simulink model "ship_5_5e"  (R2018a)
settings: Solver=VariableStepAuto  StartTime=0.0  StopTime=8000  RelTol=1e-3  EnableMultiTasking=on
values from neighbouring files (symbols this model uses):
  Kpd = sqrt(Tf^2*omegac^4+omegac^2)/K    [oppg5_3.m]    (also in oppg5_5.m = 0.8159)
  Td = T    (= 75)    [oppg5_3.m]    (also in oppg5_5.m)
  Tf = -1/(omegac*tand(130))    [oppg5_3.m]    (also in oppg5_5.m = 8.391)
libraries: simulink x1
settings Model: Creator=markh  LastModifiedBy=mariu
settings DataIOCC: LimitDataPoints=on  MaxDataPoints=100000  SaveFormat=Array  SignalLoggingSaveFormat=ModelDataLogs  SignalLoggingName=sigsOut
settings OptimizationCC: InitFltsAndDblsToZero=on  LifeSpan=inf
settings DebuggingCC: SaveWithParameterizedLinksMsg=none  UnderspecifiedInitializationDetection=Classic  MergeDetectMultiDrivingBlocksExec=none  SignalResolutionControl=TryResolveAllWithWarning  MultiTaskDSMMsg=warning  MultiTaskCondExecSysMsg=none  FcnCallInpInsideContextMsg=warning  StateNameClashWarn=warning  SFUnexpectedBacktrackingDiag=warning  SFNoUnconditionalDefaultTransitionDiag=warning  SFExecutionAtInitializationDiag=none
settings HardwareCC: ProdBitPerPointer=32  ProdBitPerSizeT=32  ProdBitPerPtrDiffT=32  ProdLargestAtomicFloat=None  ProdIntDivRoundTo=Undefined  ProdEndianess=Unspecified  ProdWordSize=32  ProdHWDeviceType=32-bit Generic  TargetUnknown=on
settings ModelReferenceCC: PropagateSignalLabelsOutOfModel=off
settings RTWCC: Description=Generic Real-Time Target
settings CodeAppCC: StateflowObjectComments=on
settings GRTTargetCC: TargetFcnLib=ansi_tfl_tmw.mat  TargetLangStandard=C89/C90 (ANSI)  GeneratePreprocessorConditionals=Disable all  CombineOutputUpdateFcns=off  GRTInterface=on
settings ConfigComp: CovMetricSettings=dw  CovHtmlReporting=on  CovSaveCumulativeToWorkspaceVar=on  CovSaveSingleToWorkspaceVar=on  CovExternalEMLEnable=off

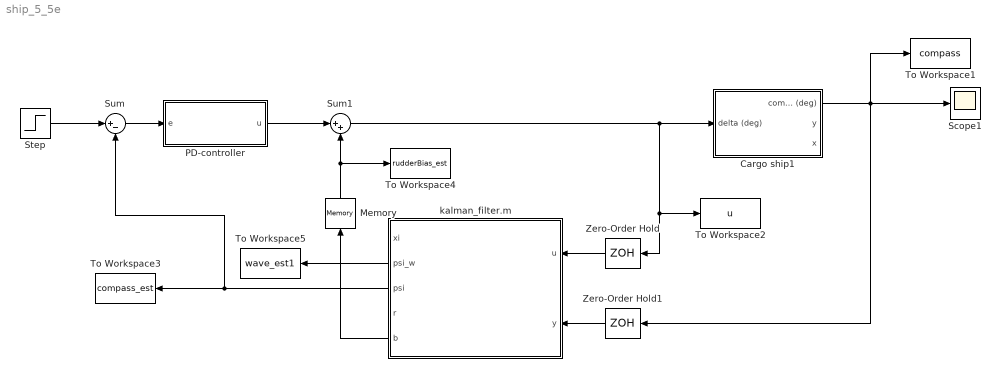
== system ship_5_5e ==
  " kalman_filter.m" : MATLAB Function  TreatAsAtomicUnit=on
  Cargo ship1 : Subsystem  mask(Simple shipmodel for a cargo ship){noise=on, current=on, logic=on}
      mask prompts: noise "measurement noise"; logic "waves"
      mask help:
      | Measurement noise:
      | 	checked = noise on
      | 	unchecked = noise off
      |
      | Current:
      | 	checked = current on
      | 	unchecked = current off
      |
      | Waves:
      | 	checked = waves on
      | 	unchecked = waves off
      |
      | Author: Jørgen Spjøtvold, 9/10-2003
      | TTK 4115 Linear system theory.
      | Modified by Jostein Bakkeheim 26/10-2006
  Memory : Memory
  PD-controller : Subsystem
  Scope1 : Scope
  Step : Step  Time=0  After=30  SampleTime=0
  Sum : Sum  Inputs=|+-
  Sum1 : Sum  Inputs=|++
  To Workspace1 : ToWorkspace  VariableName=compass  SaveFormat=Timeseries  SampleTime=-1
  To Workspace2 : ToWorkspace  VariableName=u  SaveFormat=Timeseries  SampleTime=-1
  To Workspace3 : ToWorkspace  VariableName=compass_est  SaveFormat=Timeseries  SampleTime=-1
  To Workspace4 : ToWorkspace  VariableName=rudderBias_est  SaveFormat=Timeseries  SampleTime=-1
  To Workspace5 : ToWorkspace  VariableName=wave_est1  SaveFormat=Timeseries  SampleTime=-1
  Zero-Order Hold : ZeroOrderHold  SampleTime=0.1
  Zero-Order Hold1 : ZeroOrderHold  SampleTime=0.1
  wires:
  Cargo ship1/1(compass (deg)) -> Zero-Order Hold1/1, To Workspace1/1, Scope1/1
  Sum/1 -> PD-controller/1(e)
  Zero-Order Hold1/1 -> " kalman_filter.m"/2(y)
  Zero-Order Hold/1 -> " kalman_filter.m"/1(u)
  " kalman_filter.m"/3(psi) -> Sum/2, To Workspace3/1
  PD-controller/1(u) -> Sum1/1
  Sum1/1 -> To Workspace2/1, Zero-Order Hold/1, Cargo ship1/1(delta (deg))
  " kalman_filter.m"/5(b) -> Memory/1
  Memory/1 -> To Workspace4/1, Sum1/2
  Step/1 -> Sum/1
  " kalman_filter.m"/2(psi_w) -> To Workspace5/1

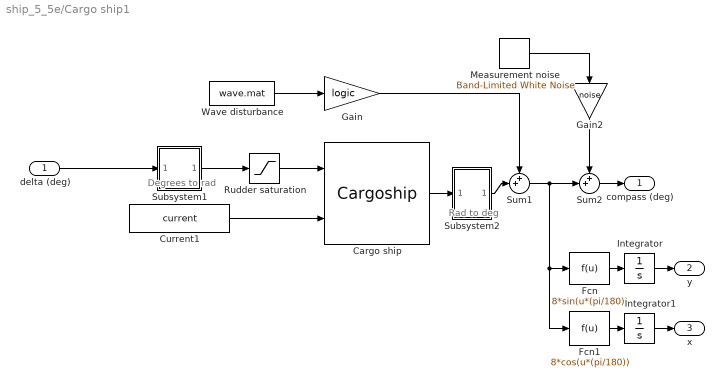
== system ship_5_5e/Cargo ship1 ==
  note: Degrees to rad
  note: Rad to deg
  delta (deg) : Inport
  Cargo ship : S-Function  FunctionName=Cargoship  SFunctionDeploymentMode=off  EnableBusSupport=off  mask(Cargo ship){}
      mask help:
      | S-function which simulates a cargo ship.
      |
      | Author: Jørgen Spjøtvold
      | 20.10-2003
      | Modified by Jostein Bakkeheim 27.10.2006
  Current1 : Constant  Value=current
  Fcn : Fcn  Expr=8*sin(u*(pi/180))
  Fcn1 : Fcn  Expr=8*cos(u*(pi/180))
  Gain : Gain  Gain=logic  SaturateOnIntegerOverflow=on  OutDataTypeStr=Inherit: Same as input  ParamDataTypeStr=Inherit: Same as input
  Gain2 : Gain  Gain=noise  SaturateOnIntegerOverflow=on  OutDataTypeStr=Inherit: Same as input  ParamDataTypeStr=Inherit: Same as input
  Integrator : Integrator
  Integrator1 : Integrator
  Measurement noise : simulink/Sources/Band-Limited White Noise  Cov=[0.001]  Ts=.5  seed=[23341]
  Rudder saturation : Saturate  UpperLimit=45*(pi/180)  LowerLimit=-45*(pi/180)
  Subsystem1 : Subsystem  mask(degrees to radians){}
      mask help: Converts degrees to radians
      mask Display: fprintf('D2R');
  Subsystem2 : Subsystem  mask(radians to degrees){}
      mask help: Converts radians to degrees
      mask Display: fprintf('R2D');
  Sum1 : Sum  Inputs=++|  SaturateOnIntegerOverflow=on
  Sum2 : Sum  Inputs=++|  SaturateOnIntegerOverflow=on
  Wave disturbance : FromFile  FileName=wave.mat  SampleTime=0
  compass (deg) : Outport
  y : Outport  Port=2
  x : Outport  Port=3
  wires:
  delta (deg)/1 -> Subsystem1/1(In1)
  Fcn/1 -> Integrator/1
  Integrator/1 -> y/1
  Fcn1/1 -> Integrator1/1
  Integrator1/1 -> x/1
  Wave disturbance/1 -> Gain/1
  Subsystem2/1(Out1) -> Sum1/2
  Gain/1 -> Sum1/1
  Sum1/1 -> Fcn/1, Fcn1/1, Sum2/2
  Cargo ship/1 -> Subsystem2/1(In1)
  Subsystem1/1(Out1) -> Rudder saturation/1
  Rudder saturation/1 -> Cargo ship/1
  Sum2/1 -> compass (deg)/1
  Measurement noise/1 -> Gain2/1
  Gain2/1 -> Sum2/1
  Current1/1 -> Cargo ship/2

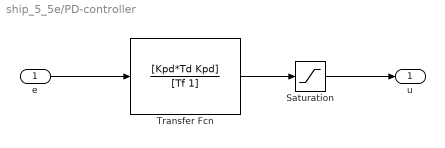
== system ship_5_5e/PD-controller ==
  e : Inport
  Saturation : Saturate  UpperLimit=35  LowerLimit=-35
  Transfer Fcn : TransferFcn  Numerator=[Kpd*Td Kpd]  Denominator=[Tf 1]
  u : Outport
  wires:
  e/1 -> Transfer Fcn/1
  Transfer Fcn/1 -> Saturation/1
  Saturation/1 -> u/1

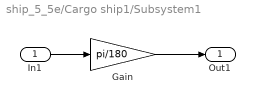
== system ship_5_5e/Cargo ship1/Subsystem1 ==
  In1 : Inport
  Gain : Gain  Gain=pi/180  SaturateOnIntegerOverflow=on  OutDataTypeStr=Inherit: Same as input  ParamDataTypeStr=Inherit: Same as input
  Out1 : Outport
  wires:
  Gain/1 -> Out1/1
  In1/1 -> Gain/1

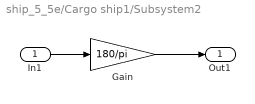
== system ship_5_5e/Cargo ship1/Subsystem2 ==
  In1 : Inport
  Gain : Gain  Gain=180/pi  SaturateOnIntegerOverflow=on  OutDataTypeStr=Inherit: Same as input  ParamDataTypeStr=Inherit: Same as input
  Out1 : Outport
  wires:
  Gain/1 -> Out1/1
  In1/1 -> Gain/1

== matlab function ship_5_5e/ kalman_filter.m ==
  settings: updateMethod=DISCRETE  sampleTime=0.1
  data: u input; xi output; y input; psi_w output; psi output; r output; b output; parameters parameter
function [xi, psi_w, psi, r, b] = kalman_filter(u,y, parameters)
    %declare variables
    persistent A B C E I Q R Pbar xbar init

    if (isempty(init))  % startingvalues (passed as a struct so we can use "from workspace")
        A = parameters.A;
        B = parameters.B;
        C = parameters.C;
        E = parameters.E;
        I = parameters.I;
        Q = parameters.Q;   %deal could make this a bit more pretty
        R = parameters.R;
        Pbar = parameters.P0bar;
        xbar = parameters.x0bar;
        init = 1;
    end

    %kalman gain
    L = (Pbar*C')*((C*Pbar*C'+R)^-1);
    %update state
    x = xbar + L*(y - C*xbar);
    % update error covariance
    P = (I - L*C)*Pbar*(I-L*C)' + L*R*(L');
    
    % estimate next state and error covariance
    xbar = A*x + B*u;
    Pbar = A*P*(A') + E*Q*(E');
    
    
    %update outputs
    xi = x(1);
    psi_w = x(2);
    psi = x(3);
    r = x(4);
    b = x(5);
end
